simulink subsystem "controlSystem"  (R2024a)
settings: Solver=VariableStepAuto  StartTime=0.0  StopTime=10.0  RelTol=1e-3
settings Model: Creator=janho  LastModifiedBy=janho

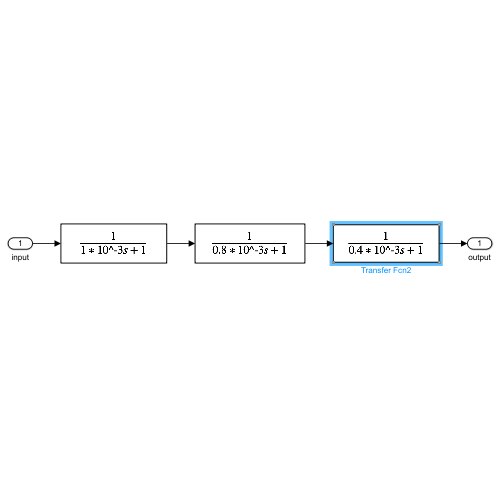
[thumbnail: Simulink's stored preview of the top-level diagram]
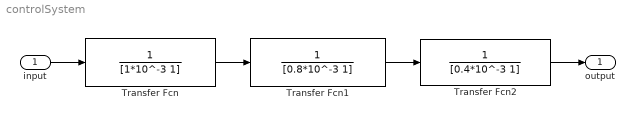
== system controlSystem ==
  input : Inport
  Transfer Fcn : TransferFcn  Denominator=[1*10^-3 1]
  Transfer Fcn1 : TransferFcn  Denominator=[0.8*10^-3 1]
  Transfer Fcn2 : TransferFcn  Denominator=[0.4*10^-3 1]
  output : Outport
  wires:
  Transfer Fcn/1 -> Transfer Fcn1/1
  Transfer Fcn1/1 -> Transfer Fcn2/1
  input/1 -> Transfer Fcn/1
  Transfer Fcn2/1 -> output/1
